simulink model "picntrl"  (R2020b)
settings: Solver=VariableStepAuto  StartTime=0.0  StopTime=10.0  RelTol=1e-3
undefined symbols (not defined in the file or in its folder): ki, kp
settings Model: Creator=intel  LastModifiedBy=intel

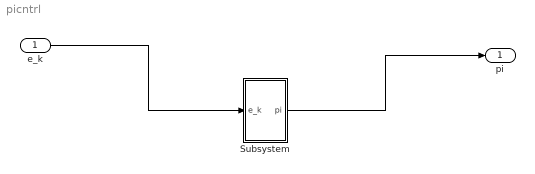
== system picntrl ==
  e_k : Inport  OutDataTypeStr=double  PortDimensions=1  SampleTime=0
  Subsystem : Subsystem
  pi : Outport  OutDataTypeStr=double  PortDimensions=1  SampleTime=0
  wires:
  e_k/1 -> Subsystem/1(e_k)
  Subsystem/1(pi) -> pi/1

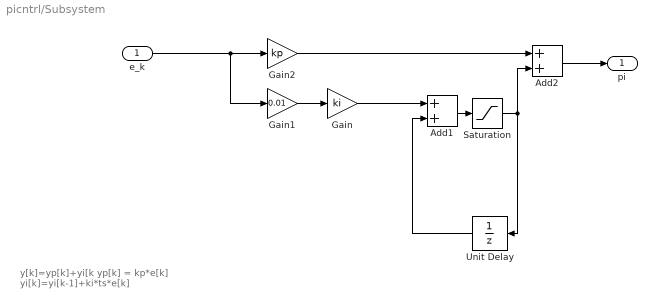
== system picntrl/Subsystem ==
  note: y[k]=yp[k]+yi[k
      | yp[k] = kp*e[k]
      | yi[k]=yi[k-1]+ki*ts*e[k]
  e_k : Inport  OutDataTypeStr=double  PortDimensions=1  SampleTime=0
  Add1 : Sum
  Add2 : Sum
  Gain : Gain  Gain=ki
  Gain1 : Gain  Gain=0.01
  Gain2 : Gain  Gain=kp
  Saturation : Saturate  UpperLimit=1  LowerLimit=-1
  Unit Delay : UnitDelay  SampleTime=-1  HasFrameUpgradeWarning=on
  pi : Outport  OutDataTypeStr=double  PortDimensions=1  SampleTime=0
  wires:
  Add2/1 -> pi/1
  Gain2/1 -> Add2/1
  Gain1/1 -> Gain/1
  Gain/1 -> Add1/1
  e_k/1 -> Gain2/1, Gain1/1
  Add1/1 -> Saturation/1
  Unit Delay/1 -> Add1/2
  Saturation/1 -> Unit Delay/1, Add2/2
